simulink model "SimForces2022a"  (R2022a)
settings: Solver=daessc  StartTime=0.0  StopTime=10  FixedStep=0.001  RelTol=1e-4
values from neighbouring files (symbols this model uses):
  Bc1_V = [0;0;0;0;0;0]    [initializeSimulationGP.m]
  D22F = [0;0;0;0;0;0]    [initializeSimulationGP.m]
  filtDV = init2ndOrderLowPassFilter(35*2*pi,1,controller.dT)    [initializeLowPassFilters.m]
  filtEnc = init2ndOrderLowPassFilter(35*2*pi,1,controller.dT)    [initializeLowPassFilters.m]
undefined symbols (not defined in the file or in its folder): aux, B11_r_B11Tc1, B11_V, B11Ftot, B12_r_B12Tc2, B12_Rot_Tc2, B12_U_Tc2, B12_V, B12Ftot, B31_r_B31B41, B31_V, B31FTot, B32_r_B32B42, B32_Rot_B42, B32_U_B42, B32_V, B32FTot, B41_r_B41Tc1, B41_V, B41FTot, B42_r_B42Tc2, B42_Rot_Tc2, B42_U_Tc2, B42_V, B42FTot, B52_r_B52P32, B52_Rot_P32, B52_U_P32, B52_V, B52Ftot, Bc1_r_Bc1B11, Bc1_r_Bc1B31, Bc1FTot, Bc2_r_Bc2B12, Bc2_r_Bc2B32, Bc2_Rot_B12, Bc2_Rot_B32, Bc2_U_B12, Bc2_U_B32, Bc2_V, Bc2Tot, controller, cyl1, cyl2, D22_V, dq1, dq11, dq12, dq2, dq21, dq22, dx1, dx2, dxt2, fc1, fc1r, fc2, fc2r, fct2, fct2r ... (+61)
libraries: sm_lib x32, nesl_utility x20
(part 3 of 7)

== system SimForces2022a/sbVDCController/sbFormAnalyticQuantities/sbRevoluteSegment2 ==
  note: Due to repeatable nature of the calculation process, all the comments in RS1 remain in RS2.
  note: Get inputs...
  note: Process data...
  note: Pass to outputs...
  q2 : Inport
  WRotXRS1 : Inport  Port=2
  velsRS1 : Inport  Port=3
  sbGeomPropRS2 : Subsystem
  sbPosVecsRS2 : Subsystem
  sbRotMatsRS2 : Subsystem
  sbUMatsRS2 : Subsystem
  sbVelsRS2 : Subsystem
  geomPropRS2 : Outport
  WRotXRS2 : Outport  Port=2
  UMatsRS2 : Outport  Port=3
  velsRS2 : Outport  Port=4
  wires:
  [velsRS2] -> velsRS2/1  "velsRS2"
  sbVelsRS2/1(velsRS2) -> [velsRS2]  "velsRS2"
  [WRotXRS1] -> sbRotMatsRS2/2(WRotXRS1)  "WRotXRS1"
  WRotXRS1/1 -> [WRotXRS1]  "WRotXRS1"
  [velsRS1] -> sbVelsRS2/3(velsRS1)  "velsRS1"
  velsRS1/1 -> [velsRS1]  "velsRS1"
  [WRotXRS2] -> WRotXRS2/1  "WRotXRS2"
  sbRotMatsRS2/2(WRotXRS2) -> [WRotXRS2]  "WRotXRS2"
  [UMatsRS2] -> UMatsRS2/1  "UMatsRS2"
  [UMatsRS2] -> sbVelsRS2/2(UMatsRS2)  "UMatsRS2"
  sbUMatsRS2/1(UMatsRS2) -> [UMatsRS2]  "UMatsRS2"
  [rotMatsRS2] -> sbUMatsRS2/2(rotMatsRS2)  "rotMatsRS2"
  [posVecsRS2] -> sbUMatsRS2/1(posVecsRS2)  "posVecsRS2"
  sbPosVecsRS2/1(posVecsRS2) -> [posVecsRS2]  "posVecsRS2"
  q2/1 -> [q2]  "q2"
  sbRotMatsRS2/1(rotMatsRS2) -> [rotMatsRS2]  "rotMatsRS2"
  [geomPropRS2] -> geomPropRS2/1  "geomPropRS2"
  [q2] -> sbGeomPropRS2/1(q2)  "q2"
  sbGeomPropRS2/1(geomPropRS2) -> [geomPropRS2]  "geomPropRS2"
  [geomPropRS2] -> sbPosVecsRS2/1(geomPropRS2)  "geomPropRS2"
  [geomPropRS2] -> sbRotMatsRS2/1(geomPropRS2)  "geomPropRS2"
  [geomPropRS2] -> sbVelsRS2/1(geomPropRS2)  "geomPropRS2"

== system SimForces2022a/sbVDCController/sbFormTotalRequiredForces/sbTotalRequiredForcesPS2 ==
  note: Form new buses...
  note: Pass to outputs...
  note: Process data...
  note: Get inputs...
  note: Select from existing buses...
  note: Calculate total forces in the prismatic segment 2 (PS2).
  velsX : Inport
  WRotX : Inport  Port=2
  Bus Creator1 : BusCreator  Inputs=P22FTot,B52Ftot,P32FTot
  Bus Selector2 : BusSelector  OutputSignals=WRotXRS2.W_Rot_P22,WRotXPS2.W_Rot_B52,WRotXPS2.W_Rot_P32
  Bus Selector3 : BusSelector  OutputSignals=velsRS2.P22_V,velsPS2.B52_V,velsPS2.P32_V
  Constant : Constant  Value=update.thetaB52rNominal
  Constant1 : Constant  Value=update.thetaP22rNominal
  Constant2 : Constant  Value=update.thetaP32rNominal
  Product1 : Product  Multiplication=Matrix(*)
  Product2 : Product  Multiplication=Matrix(*)
  Product3 : Product  Multiplication=Matrix(*)
  Transpose : Math  Operator=transpose
  Transpose1 : Math  Operator=transpose
  Transpose2 : Math  Operator=transpose
  regressorYB52r : MATLAB Function  TreatAsAtomicUnit=on
  regressorYP22r : MATLAB Function  TreatAsAtomicUnit=on
  regressorYP32r : MATLAB Function  TreatAsAtomicUnit=on
  sbFilteredVelocityDerivativeB52 : Subsystem
  sbFilteredVelocityDerivativeP22 : Subsystem
  sbFilteredVelocityDerivativeP32 : Subsystem
  FTotRS2 : Outport
  wires:
  [B52FTot] -> Bus Creator1/2  "B52Ftot"
  Bus Selector3/3 -> [P32V]  "<P32_V>"
  velsX/1 -> [velsX]  "velsX"
  Bus Selector3/2 -> [B52V]  "<B52_V>"
  Bus Selector2/3 -> [WRotP32]  "<W_Rot_P32>"
  WRotX/1 -> [WRotX]  "WRotX"
  [velsX] -> Bus Selector3/1  "velsX"
  Bus Selector2/2 -> [WRotB52]  "<W_Rot_B52>"
  [FTotRS2] -> FTotRS2/1  "FTotRS2"
  [P32FTot] -> Bus Creator1/3  "P32FTot"
  [P22FTot] -> Bus Creator1/1  "P22FTot"
  [WRotX] -> Bus Selector2/1  "WRotX"
  Bus Selector2/1 -> [WRotP22]  "<W_Rot_P22>"
  Bus Selector3/1 -> [P22V]  "<P22_V>"
  Bus Creator1/1 -> [FTotRS2]  "FTotRS2"
  [WRotP32] -> Transpose2/1  "W_Rot_P32"
  [WRotB52] -> Transpose1/1  "W_Rot_B52"
  regressorYP32r/1(YP32r) -> Product3/1  "YP32r"
  regressorYB52r/1(YB52r) -> Product2/1  "YB52r"
  [WRotP22] -> Transpose/1  "W_Rot_P22"
  [P32V] -> sbFilteredVelocityDerivativeP32/1(u)  "P32V"
  Transpose1/1 -> regressorYB52r/3(B52_Rot_W)  "B52_Rot_W"
  Transpose2/1 -> regressorYP32r/3(P32_Rot_W)  "P32_Rot_W"
  sbFilteredVelocityDerivativeP22/1(du) -> regressorYP22r/2(P22dV)  "P22dV"
  Product1/1 -> [P22FTot]  "P22FTot"
  Product3/1 -> [P32FTot]  "P32FTot"
  Product2/1 -> [B52FTot]  "B52FTot"
  sbFilteredVelocityDerivativeB52/1(du) -> regressorYB52r/2(B52dV)  "B52dV"
  [B52V] -> sbFilteredVelocityDerivativeB52/1(u)  "B52V"
  sbFilteredVelocityDerivativeP32/1(du) -> regressorYP32r/2(P32dV)  "P32dV"
  Transpose/1 -> regressorYP22r/3(P22_Rot_W)  "P22_Rot_W"
  [P22V] -> sbFilteredVelocityDerivativeP22/1(u)  "P22V"
  regressorYP22r/1(YP22r) -> Product1/1  "YP22r"
  Constant/1 -> Product2/2  "thetaB52rNominal"
  Constant1/1 -> Product1/2  "thetaP22rNominal"
  Constant2/1 -> Product3/2  "thetaP32rNominal"
  [P32V] -> regressorYP32r/1(P32V)  "P32V"
  [B52V] -> regressorYB52r/1(B52V)  "B52V"
  [P22V] -> regressorYP22r/1(P22V)  "P22V"

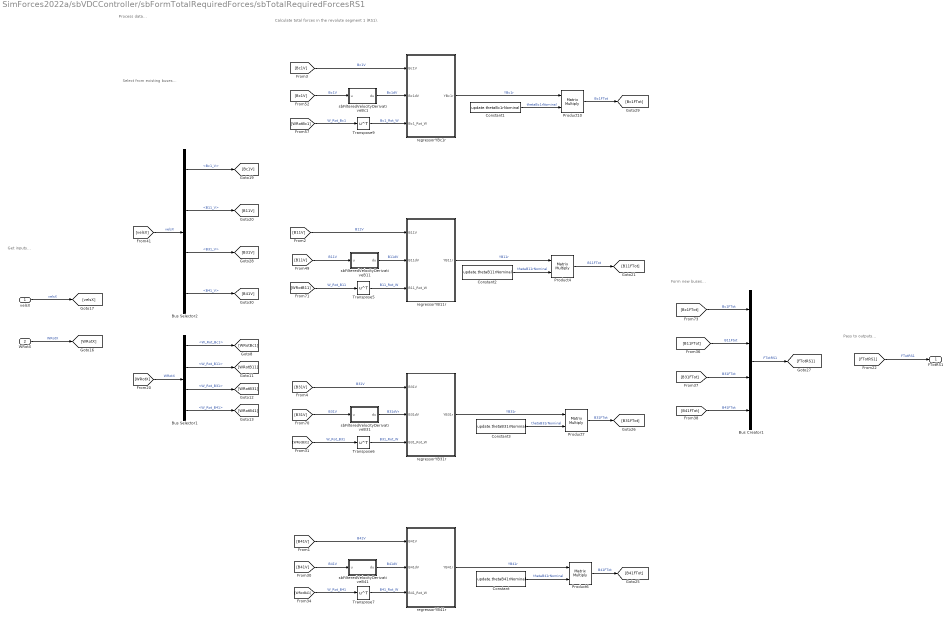
== system SimForces2022a/sbVDCController/sbFormTotalRequiredForces/sbTotalRequiredForcesRS1 ==
  note: Select from existing buses...
  note: Process data...
  note: Get inputs...
  note: Pass to outputs...
  note: Calculate total forces in the revolute segment 1 (RS1).
  note: Form new buses...
  velsX : Inport
  WRotX : Inport  Port=2
  Bus Creator1 : BusCreator  Inputs=Bc1FTot,B11Ftot,B31FTot,B41FTot
  Bus Selector1 : BusSelector  OutputSignals=WRotXRS1.W_Rot_Bc1,WRotXRS1.W_Rot_B11,WRotXRS1.W_Rot_B31,WRotXRS1.W_Rot_B41
  Bus Selector2 : BusSelector  OutputSignals=velsRS1.Bc1_V,velsRS1.B11_V,velsRS1.B31_V,velsRS1.B41_V
  Constant : Constant  Value=update.thetaB41rNominal
  Constant1 : Constant  Value=update.thetaBc1rNominal
  Constant2 : Constant  Value=update.thetaB11rNominal
  Constant3 : Constant  Value=update.thetaB31rNominal
  Product{4,6..7,10} (4 alike) : Product  Multiplication=Matrix(*)
  Transpose{5..7,9} (4 alike) : Math  Operator=transpose
  regressorYB11r : MATLAB Function  TreatAsAtomicUnit=on
  regressorYB31r : MATLAB Function  TreatAsAtomicUnit=on
  regressorYB41r : MATLAB Function  TreatAsAtomicUnit=on
  regressorYBc1r : MATLAB Function  TreatAsAtomicUnit=on
  sbFilteredVelocityDerivativeB11 : Subsystem
  sbFilteredVelocityDerivativeB31 : Subsystem
  sbFilteredVelocityDerivativeB41 : Subsystem
  sbFilteredVelocityDerivativeBc1 : Subsystem
  FTotRS1 : Outport
  wires:
  [FTotRS1] -> FTotRS1/1  "FTotRS1"
  velsX/1 -> [velsX]  "velsX"
  [WRotX] -> Bus Selector1/1  "WRotX"
  WRotX/1 -> [WRotX]  "WRotX"
  Bus Selector1/4 -> [WRotB41]  "<W_Rot_B41>"
  Bus Selector1/2 -> [WRotB11]  "<W_Rot_B11>"
  Bus Selector1/1 -> [WRotBc1]  "<W_Rot_Bc1>"
  Bus Selector1/3 -> [WRotB31]  "<W_Rot_B31>"
  regressorYB31r/1(YB31r) -> Product7/1  "YB31r"
  sbFilteredVelocityDerivativeB31/1(du) -> regressorYB31r/2(B31dV)  "B31dVr"
  [velsX] -> Bus Selector2/1  "velsX"
  sbFilteredVelocityDerivativeB41/1(du) -> regressorYB41r/2(B41dV)  "B41dV"
  Bus Creator1/1 -> [FTotRS1]  "FTotRS1"
  Product10/1 -> [Bc1FTot]  "Bc1FTot"
  [Bc1FTot] -> Bus Creator1/1  "Bc1FTot"
  [WRotB31] -> Transpose6/1  "W_Rot_B31"
  [B41FTot] -> Bus Creator1/4  "B41FTot"
  Bus Selector2/1 -> [Bc1V]  "<Bc1_V>"
  [B31FTot] -> Bus Creator1/3  "B31FTot"
  [WRotBc1] -> Transpose9/1  "W_Rot_Bc1"
  Transpose5/1 -> regressorYB11r/3(B11_Rot_W)  "B11_Rot_W"
  [WRotB11] -> Transpose5/1  "W_Rot_B11"
  Bus Selector2/2 -> [B11V]  "<B11_V>"
  Bus Selector2/4 -> [B41V]  "<B41_V>"
  regressorYBc1r/1(YBc1r) -> Product10/1  "YBc1r"
  regressorYB11r/1(YB11r) -> Product4/1  "YB11r"
  regressorYB41r/1(YB41r) -> Product6/1  "YB41r"
  [WRotB41] -> Transpose7/1  "W_Rot_B41"
  sbFilteredVelocityDerivativeB11/1(du) -> regressorYB11r/2(B11dV)  "B11dV"
  [Bc1V] -> sbFilteredVelocityDerivativeBc1/1(u)  "Bc1V"
  Transpose7/1 -> regressorYB41r/3(B41_Rot_W)  "B41_Rot_W"
  Transpose9/1 -> regressorYBc1r/3(Bc1_Rot_W)  "Bc1_Rot_W"
  [B11FTot] -> Bus Creator1/2  "B11Ftot"
  Product6/1 -> [B41FTot]  "B41FTot"
  Bus Selector2/3 -> [B31V]  "<B31_V>"
  [Bc1V] -> regressorYBc1r/1(Bc1V)  "Bc1V"
  sbFilteredVelocityDerivativeBc1/1(du) -> regressorYBc1r/2(Bc1dV)  "Bc1dV"
  Transpose6/1 -> regressorYB31r/3(B31_Rot_W)  "B31_Rot_W"
  Product4/1 -> [B11FTot]  "B11FTot"
  Product7/1 -> [B31FTot]  "B31FTot"
  Constant/1 -> Product6/2  "thetaB41rNominal"
  Constant3/1 -> Product7/2  "thetaB31rNominal"
  Constant2/1 -> Product4/2  "thetaB11rNominal"
  Constant1/1 -> Product10/2  "thetaBc1rNominal"
  [B41V] -> sbFilteredVelocityDerivativeB41/1(u)  "B41V"
  [B41V] -> regressorYB41r/1(B41V)  "B41V"
  [B11V] -> sbFilteredVelocityDerivativeB11/1(u)  "B11V"
  [B11V] -> regressorYB11r/1(B11V)  "B11V"
  [B31V] -> sbFilteredVelocityDerivativeB31/1(u)  "B31V"
  [B31V] -> regressorYB31r/1(B31V)  "B31V"

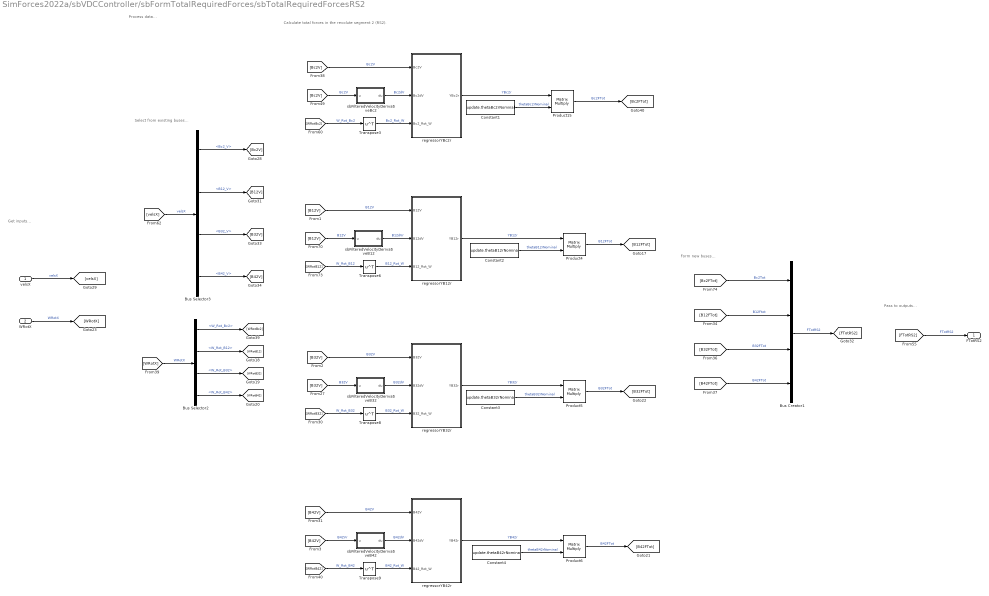
== system SimForces2022a/sbVDCController/sbFormTotalRequiredForces/sbTotalRequiredForcesRS2 ==
  note: Form new buses...
  note: Calculate total forces in the revolute segment 2 (RS2).
  note: Select from existing buses...
  note: Process data...
  note: Pass to outputs...
  note: Get inputs...
  velsX : Inport
  WRotX : Inport  Port=2
  Bus Creator1 : BusCreator  Inputs=Bc2Tot,B12Ftot,B32FTot,B42FTot
  Bus Selector2 : BusSelector  OutputSignals=WRotXRS1.W_Rot_Bc2,WRotXRS2.W_Rot_B12,WRotXRS2.W_Rot_B32,WRotXRS2.W_Rot_B42
  Bus Selector3 : BusSelector  OutputSignals=velsRS2.Bc2_V,velsRS2.B12_V,velsRS2.B32_V,velsRS2.B42_V
  Constant1 : Constant  Value=update.thetaBc2rNominal
  Constant2 : Constant  Value=update.thetaB12rNominal
  Constant3 : Constant  Value=update.thetaB32rNominal
  Constant4 : Constant  Value=update.thetaB42rNominal
  Product{4..6,15} (4 alike) : Product  Multiplication=Matrix(*)
  Transpose{3,6,8..9} (4 alike) : Math  Operator=transpose
  regressorYB12r : MATLAB Function  TreatAsAtomicUnit=on
  regressorYB32r : MATLAB Function  TreatAsAtomicUnit=on
  regressorYB42r : MATLAB Function  TreatAsAtomicUnit=on
  regressorYBc2r : MATLAB Function  TreatAsAtomicUnit=on
  sbFilteredVelocityDerivativeB12 : Subsystem
  sbFilteredVelocityDerivativeB32 : Subsystem
  sbFilteredVelocityDerivativeB42 : Subsystem
  sbFilteredVelocityDerivativeBc2 : Subsystem
  FTotRS2 : Outport
  wires:
  Bus Selector3/1 -> [Bc2V]  "<Bc2_V>"
  Bus Selector2/1 -> [WRotBc2]  "<W_Rot_Bc2>"
  Bus Creator1/1 -> [FTotRS2]  "FTotRS2"
  [B32FTot] -> Bus Creator1/3  "B32FTot"
  [WRotX] -> Bus Selector2/1  "WRotX"
  [FTotRS2] -> FTotRS2/1  "FTotRS2"
  [B42FTot] -> Bus Creator1/4  "B42FTot"
  [Bc2FTot] -> Bus Creator1/1  "Bc2Tot"
  Product5/1 -> [B32FTot]  "B32FTot"
  Bus Selector2/2 -> [WRotB12]  "<W_Rot_B12>"
  Bus Selector2/4 -> [WRotB42]  "<W_Rot_B42>"
  Transpose6/1 -> regressorYB12r/3(B12_Rot_W)  "B12_Rot_W"
  [B32V] -> sbFilteredVelocityDerivativeB32/1(u)  "B32V"
  [WRotB32] -> Transpose8/1  "W_Rot_B32"
  sbFilteredVelocityDerivativeB32/1(du) -> regressorYB32r/2(B32dV)  "B32dV"
  Product15/1 -> [Bc2FTot]  "Bc2FTot"
  [B42V] -> sbFilteredVelocityDerivativeB42/1(u)  "B42Vr"
  Transpose9/1 -> regressorYB42r/3(B42_Rot_W)  "B42_Rot_W"
  Product6/1 -> [B42FTot]  "B42FTot"
  regressorYB32r/1(YB32r) -> Product5/1  "YB32r"
  regressorYBc2r/1(YBc2r) -> Product15/1  "YBc2r"
  regressorYB12r/1(YB12r) -> Product4/1  "YB12r"
  [velsX] -> Bus Selector3/1  "velsX"
  [WRotB42] -> Transpose9/1  "W_Rot_B42"
  regressorYB42r/1(YB42r) -> Product6/1  "YB42r"
  Bus Selector3/4 -> [B42V]  "<B42_V>"
  WRotX/1 -> [WRotX]  "WRotX"
  Transpose8/1 -> regressorYB32r/3(B32_Rot_W)  "B32_Rot_W"
  Bus Selector2/3 -> [WRotB32]  "<W_Rot_B32>"
  [WRotBc2] -> Transpose3/1  "W_Rot_Bc2"
  sbFilteredVelocityDerivativeBc2/1(du) -> regressorYBc2r/2(Bc2dV)  "Bc2dV"
  Product4/1 -> [B12FTot]  "B12FTot"
  [B32V] -> regressorYB32r/1(B32V)  "B32V"
  [WRotB12] -> Transpose6/1  "W_Rot_B12"
  sbFilteredVelocityDerivativeB42/1(du) -> regressorYB42r/2(B42dV)  "B42dV"
  sbFilteredVelocityDerivativeB12/1(du) -> regressorYB12r/2(B12dV)  "B12dVr"
  Bus Selector3/2 -> [B12V]  "<B12_V>"
  Bus Selector3/3 -> [B32V]  "<B32_V>"
  [Bc2V] -> sbFilteredVelocityDerivativeBc2/1(u)  "Bc2V"
  velsX/1 -> [velsX]  "velsX"
  Transpose3/1 -> regressorYBc2r/3(Bc2_Rot_W)  "Bc2_Rot_W"
  [B12FTot] -> Bus Creator1/2  "B12Ftot"
  Constant4/1 -> Product6/2  "thetaB42rNominal"
  Constant3/1 -> Product5/2  "thetaB32rNominal"
  Constant2/1 -> Product4/2  "thetaB12rNominal"
  [Bc2V] -> regressorYBc2r/1(Bc2V)  "Bc2V"
  Constant1/1 -> Product15/2  "thetaBc2rNominal"
  [B12V] -> sbFilteredVelocityDerivativeB12/1(u)  "B12V"
  [B12V] -> regressorYB12r/1(B12V)  "B12V"
  [B42V] -> regressorYB42r/1(B42V)  "B42V"

== system SimForces2022a/sbVDCController/sbFormAnalyticQuantities/sbPrismaticSegment2/sbGeomPropPS2 ==
  note: Get inputs...
  note: Process data...
  note: Pass to outputs...
  xt2 : Inport
  Bus Creator : BusCreator  Inputs=xt2,dxt2
  sbDiscreteDerivative : Subsystem
  geomPropPS2 : Outport
  wires:
  xt2/1 -> [xt2]
  [xt2] -> sbDiscreteDerivative/1(u)  "xt2"
  sbDiscreteDerivative/1(du/dt) -> [dxt2]  "dxt2"
  [xt2] -> Bus Creator/1  "xt2"
  [dxt2] -> Bus Creator/2  "dxt2"
  Bus Creator/1 -> [geomPropPS2]  "geomPropPS2"
  [geomPropPS2] -> geomPropPS2/1  "geomPropPS2"

== system SimForces2022a/sbVDCController/sbFormAnalyticQuantities/sbPrismaticSegment2/sbPosVecsPS2 ==
  note: Get inputs...
  note: Process data...
  note: Pass to outputs...
  xt2 : Inport
  Bus Creator : BusCreator  Inputs=P22_r_P22B52,B52_r_B52P32,P32_r_P32D22
  Constant : Constant  Value=posVec.B52_r_B52P32
  Constant1 : Constant  Value=posVec.P32_r_P32D22
  P22_r_P22B52 : MATLAB Function  TreatAsAtomicUnit=on
  posVecsPS2 : Outport
  wires:
  [rP32D22] -> Bus Creator/3  "P32_r_P32D22"
  Constant1/1 -> [rP32D22]  "P32_r_P32D22"
  [PosVecsS2P] -> posVecsPS2/1
  Bus Creator/1 -> [PosVecsS2P]
  [rB52P32] -> Bus Creator/2  "B52_r_B52P32"
  [rP22B52] -> Bus Creator/1  "P22_r_P22B52"
  Constant/1 -> [rB52P32]  "B52_r_B52P32"
  P22_r_P22B52/1(P22_r_P22B52) -> [rP22B52]  "P22_r_P22B52"
  [xt2] -> P22_r_P22B52/1(xt2)
  xt2/1 -> [xt2]

== system SimForces2022a/sbVDCController/sbFormAnalyticQuantities/sbPrismaticSegment2/sbRotMatsPS2 ==
  note: Process data...
  note: Get inputs...
  note: Pass to outputs...
  WRotXRS2 : Inport
  Bus Creator1 : BusCreator  Inputs=W_Rot_B52,W_Rot_P32,W_Rot_D22
  Bus Creator2 : BusCreator  Inputs=P22_Rot_B52,B52_Rot_P32,P32_Rot_D22
  Bus Selector : BusSelector  OutputSignals=W_Rot_P22
  Constant : Constant  Value=rotMat.P22_Rot_B52
  Constant1 : Constant  Value=rotMat.B52_Rot_P32
  Constant2 : Constant  Value=rotMat.P32_Rot_D22
  Product : Product  Multiplication=Matrix(*)
  Product1 : Product  Multiplication=Matrix(*)
  Product2 : Product  Multiplication=Matrix(*)
  rotMatsPS2 : Outport
  WRotXPS2 : Outport  Port=2
  wires:
  Product2/1 -> [WRotD22]
  [WRotD22] -> Bus Creator1/3  "W_Rot_D22"
  [P32RotD22] -> Bus Creator2/3  "P32_Rot_D22"
  [P32RotD22] -> Product2/2
  [WRotP32] -> Product2/1
  Constant2/1 -> [P32RotD22]  "P32_Rot_D22"
  [rotMatsPS2] -> rotMatsPS2/1  "rotMatsPS2"
  [WRotXPS2] -> WRotXPS2/1  "WRotXPS2"
  Bus Creator1/1 -> [WRotXPS2]  "WRotXPS2"
  Bus Creator2/1 -> [rotMatsPS2]  "rotMatsPS2"
  [WRotXRS2] -> Bus Selector/1  "WRotXRS2"
  WRotXRS2/1 -> [WRotXRS2]  "WRotXRS2"
  Bus Selector/1 -> [WRotP22]  "<W_Rot_P22>"
  [P22RotB52] -> Bus Creator2/1  "P22_Rot_B52"
  [B52RotP32] -> Bus Creator2/2  "B52_Rot_P32"
  [WRotP32] -> Bus Creator1/2  "W_Rot_P32"
  [WRotB52] -> Bus Creator1/1  "W_Rot_B52"
  Product1/1 -> [WRotP32]
  [WRotB52] -> Product1/1
  [B52RotP32] -> Product1/2
  Product/1 -> [WRotB52]
  [P22RotB52] -> Product/2
  [WRotP22] -> Product/1
  Constant1/1 -> [B52RotP32]  "B52_Rot_P32"
  Constant/1 -> [P22RotB52]  "P22_Rot_B52"

== system SimForces2022a/sbVDCController/sbFormAnalyticQuantities/sbPrismaticSegment2/sbUMatsPS2 ==
  note: Get inputs...
  note: Process data...
  note: Pass to outputs...
  posVecsPS2 : Inport
  rotMatsPS2 : Inport  Port=2
  B52_U_P32 : MATLAB Function  TreatAsAtomicUnit=on
  Bus Creator : BusCreator  Inputs=P22_U_B52,B52_U_P32,P32_U_D22
  Bus Selector : BusSelector  OutputSignals=P22_r_P22B52,B52_r_B52P32,P32_r_P32D22
  Bus Selector1 : BusSelector  OutputSignals=P22_Rot_B52,B52_Rot_P32,P32_Rot_D22
  P22_U_B52 : MATLAB Function  TreatAsAtomicUnit=on
  P32_U_D22 : MATLAB Function  TreatAsAtomicUnit=on
  UMatsPS2 : Outport
  wires:
  [P32UD22] -> Bus Creator/3  "P32_U_D22"
  P32_U_D22/1(P32_U_D22) -> [P32UD22]  "P32_U_D22"
  [P32RotD22] -> P32_U_D22/2(P32_Rot_D22)
  [rP32D22] -> P32_U_D22/1(P32_r_P32D22)
  Bus Selector/3 -> [rP32D22]  "<P32_r_P32D22>"
  Bus Selector1/3 -> [P32RotD22]  "<P32_Rot_D22>"
  Bus Creator/1 -> [UMatsS2P]
  [UMatsS2P] -> UMatsPS2/1
  [B52UP32] -> Bus Creator/2  "B52_U_P32"
  [P22UB52] -> Bus Creator/1  "P22_U_B52"
  B52_U_P32/1(B52_U_P32) -> [B52UP32]  "B52_U_P32"
  [rB52P32] -> B52_U_P32/1(B52_r_B52B32)
  [B52RotP32] -> B52_U_P32/2(B52_Rot_B32)
  P22_U_B52/1(P22_U_B52) -> [P22UB52]  "P22_U_B52"
  [P22RotB52] -> P22_U_B52/2(P22_Rot_B52)
  [rP22B52] -> P22_U_B52/1(P22_r_P22B52)
  Bus Selector/2 -> [rB52P32]  "<B52_r_B52P32>"
  Bus Selector1/2 -> [B52RotP32]  "<B52_Rot_P32>"
  Bus Selector1/1 -> [P22RotB52]  "<P22_Rot_B52>"
  Bus Selector/1 -> [rP22B52]  "<P22_r_P22B52>"
  [RotMatsS2P] -> Bus Selector1/1
  [PosVecsS2P] -> Bus Selector/1
  rotMatsPS2/1 -> [RotMatsS2P]
  posVecsPS2/1 -> [PosVecsS2P]

== system SimForces2022a/sbVDCController/sbFormAnalyticQuantities/sbPrismaticSegment2/sbVelsPS2 ==
  note: Get inputs...
  note: Process data...
  note: Pass to outputs...
  geomPropPS2 : Inport
  UMatsPS2 : Inport  Port=2
  velsRS2 : Inport  Port=3
  Bus Creator : BusCreator  Inputs=B52_V,P32_V,D22_V
  Bus Selector : BusSelector  OutputSignals=dxt2
  Bus Selector1 : BusSelector  OutputSignals=P22_V
  Bus Selector2 : BusSelector  OutputSignals=P22_U_B52,B52_U_P32,P32_U_D22
  Gain : Gain  Gain=aux.xf
  Product : Product  Multiplication=Matrix(*)
  Product1 : Product  Multiplication=Matrix(*)
  Product2 : Product  Multiplication=Matrix(*)
  Sum : Sum  Inputs=|++
  Transpose : Math  Operator=transpose
  Transpose1 : Math  Operator=transpose
  Transpose2 : Math  Operator=transpose
  velsPS2 : Outport
  wires:
  [D22V] -> Bus Creator/3  "D22_V"
  Product2/1 -> [D22V]
  Transpose2/1 -> Product2/1
  [P32UG] -> Transpose2/1
  [P32V] -> Product2/2
  Bus Selector2/3 -> [P32UG]  "<P32_U_D22>"
  [velsPS2] -> velsPS2/1  "velsPS2"
  Bus Creator/1 -> [velsPS2]  "velsPS2"
  [B52V] -> Bus Creator/1  "B52_V"
  [P32V] -> Bus Creator/2  "P32_V"
  Product1/1 -> [P32V]
  [B52UP32] -> Transpose1/1
  Transpose1/1 -> Product1/1
  [B52V] -> Product1/2
  Transpose/1 -> Product/1
  [P22UB52] -> Transpose/1
  [P22V] -> Product/2
  Product/1 -> Sum/2
  Gain/1 -> Sum/1
  Bus Selector2/2 -> [B52UP32]  "<B52_U_P32>"
  Bus Selector2/1 -> [P22UB52]  "<P22_U_B52>"
  [UMatsS2P] -> Bus Selector2/1  "UMatsPS2"
  Sum/1 -> [B52V]
  [dxt2] -> Gain/1
  Bus Selector1/1 -> [P22V]  "<P22_V>"
  UMatsPS2/1 -> [UMatsS2P]  "UMatsPS2"
  [velsRS2] -> Bus Selector1/1  "velsRS2"
  velsRS2/1 -> [velsRS2]  "velsRS2"
  geomPropPS2/1 -> [geomPropPS2]  "geomPropPS2"
  [geomPropPS2] -> Bus Selector/1  "geomPropPS2"
  Bus Selector/1 -> [dxt2]  "<dxt2>"

== system SimForces2022a/sbVDCController/sbFormAnalyticQuantities/sbRevoluteSegment1/sbGeomPropRS1 ==
  note: Calculate lift piston velocity per (21).
  note: Calculate angle q1 derivative numerically.
  note: Calculate q12 angle value per (20).
  note: Calculate q11 angle value per (19).
  note: Calculate lift piston stroke per (18).
  note: Create new buses...
  note: Process data...
  note: Pass to outputs...
  note: Get inputs...
  note: Calculate q11 angle velocity per (22).
  note: Calculate q12 angle velocity per (23).
  q1 : Inport
  Bus Creator : BusCreator  Inputs=q1,x1,q11,q12,dq1,dx1,dq11,dq12
  sbLiftPistonStroke : Subsystem
  sbLiftPistonVelocity : Subsystem
  sbq11AngleValue : Subsystem
  sbq11AngleVelocity : Subsystem
  sbq12AngleRate : Subsystem
  sbq12AngleValue : Subsystem
  sbq1AngleRate : Subsystem
  geomPropRS1 : Outport
  wires:
  [q12] -> sbq12AngleRate/2(q12)  "q12"
  [x1] -> sbq12AngleRate/1(x1)  "x1"
  [dx1] -> sbq12AngleRate/3(dx1)  "dx1"
  sbq12AngleRate/1(dq12) -> [dq12]  "dq12"
  sbq11AngleVelocity/1(dq11) -> [dq11]  "dq11"
  [q11] -> sbq11AngleVelocity/2(q11)  "q11"
  [x1] -> sbq11AngleVelocity/1(x1)  "x1"
  [dx1] -> sbq11AngleVelocity/3(dx1)  "dx1"
  sbLiftPistonVelocity/1(dx1) -> [dx1]  "dx1"
  [q1] -> sbLiftPistonVelocity/3(q1)  "q1"
  [x1] -> sbLiftPistonVelocity/2(x1)  "x1"
  [dq1] -> sbLiftPistonVelocity/1(dq1)  "dq1"
  sbq1AngleRate/1(dq1) -> [dq1]  "dq1"
  [q1] -> sbq1AngleRate/1(q1)  "q1"
  [geomPropRS1] -> geomPropRS1/1  "geomPropRS1"
  Bus Creator/1 -> [geomPropRS1]  "geomPropRS1"
  [dq11] -> Bus Creator/7  "dq11"
  [dq12] -> Bus Creator/8  "dq12"
  [dx1] -> Bus Creator/6  "dx1"
  [q11] -> Bus Creator/3  "q11"
  sbq11AngleValue/1(q11) -> [q11]  "q11"
  [x1] -> Bus Creator/2  "x1"
  [q1] -> Bus Creator/1  "q1"
  [q12] -> Bus Creator/4  "q12"
  sbq12AngleValue/1(q12) -> [q12]  "q12"
  [dq1] -> Bus Creator/5  "dq1"
  [x1] -> sbq12AngleValue/1(x1)  "x1"
  [x1] -> sbq11AngleValue/1(x1)  "x1"
  sbLiftPistonStroke/1(x1) -> [x1]  "x1"
  [q1] -> sbLiftPistonStroke/1(q1)  "q1"
  q1/1 -> [q1]  "q1"

== system SimForces2022a/sbVDCController/sbFormAnalyticQuantities/sbRevoluteSegment1/sbPosVecsRS1 ==
  note: Get inputs...
  note: Form time-varying position vectors...
  note: Process data...
  note: Create new buses...
  note: Pass to outputs...
  note: Select from existing buses...
  geomPropRS1 : Inport
  B11_r_B11Tc1 : Constant  Value=posVec.B11_r_B11Tc1
  B31_r_B31B41 : MATLAB Function  TreatAsAtomicUnit=on
  B41_r_B41Tc1 : Constant  Value=posVec.B41_r_B41Tc1
  Bc1_r_Bc1B11 : Constant  Value=posVec.Bc1_r_Bc1B11
  Bc1_r_Bc1B31 : Constant  Value=posVec.Bc1_r_Bc1B31
  Bus Creator : BusCreator  Inputs=Tc1_r_Tc1Bc2,B41_r_B41Tc1,B31_r_B31B41,Bc1_r_Bc1B31,B11_r_B11Tc1,Bc1_r_Bc1B11,W_r_WBc1
  Bus Selector : BusSelector  OutputSignals=x1
  Tc1_r_Tc1Bc2 : Constant  Value=posVec.Tc1_r_Tc1Bc2
  W_r_WBc1 : Constant  Value=posVec.W_r_WBc1
  posVecsRS1 : Outport
  wires:
  W_r_WBc1/1 -> [rWBc1]  "W_r_WBc1"
  [rWBc1] -> Bus Creator/7  "W_r_WBc1"
  [posVecsRS1] -> posVecsRS1/1  "posVecsRS1"
  [x1] -> B31_r_B31B41/1(x1)  "x1"
  Bus Selector/1 -> [x1]  "<x1>"
  [rBc1B11] -> Bus Creator/6  "Bc1_r_Bc1B11"
  [rB11Tc1] -> Bus Creator/5  "B11_r_B11Tc1"
  [rBc1B31] -> Bus Creator/4  "Bc1_r_Bc1B31"
  Bc1_r_Bc1B11/1 -> [rBc1B11]  "Bc1_r_Bc1B11"
  B11_r_B11Tc1/1 -> [rB11Tc1]  "B11_r_B11Tc1"
  Bc1_r_Bc1B31/1 -> [rBc1B31]  "Bc1_r_Bc1B31"
  [rB31B41] -> Bus Creator/3  "B31_r_B31B41"
  B31_r_B31B41/1(B31_r_B31B41) -> [rB31B41]  "B31_r_B31B41"
  [rB41Tc1] -> Bus Creator/2  "B41_r_B41Tc1"
  B41_r_B41Tc1/1 -> [rB41Tc1]  "B41_r_B41Tc1"
  [rTc1Bc2] -> Bus Creator/1  "Tc1_r_Tc1Bc2"
  Tc1_r_Tc1Bc2/1 -> [rTc1Bc2]  "Tc1_r_Tc1Bc2"
  [geomPropRS1] -> Bus Selector/1  "geomPropRS1"
  geomPropRS1/1 -> [geomPropRS1]  "geomPropRS1"
  Bus Creator/1 -> [posVecsRS1]  "posVecsRS1"

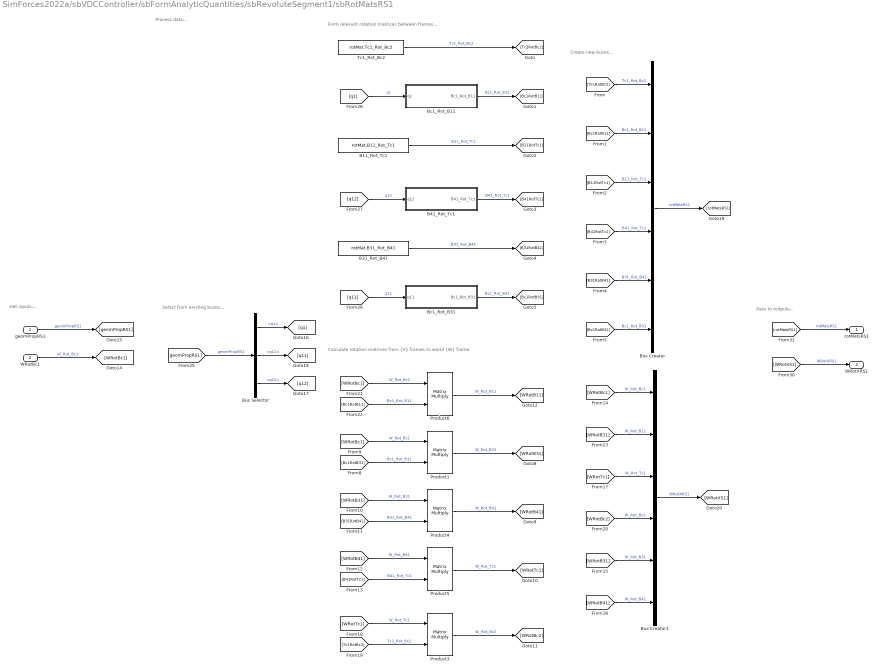
== system SimForces2022a/sbVDCController/sbFormAnalyticQuantities/sbRevoluteSegment1/sbRotMatsRS1 ==
  note: Calculate rotation matrices from {X} frames to world {W} frame
  note: Form relevant rotation matrices between frames...
  note: Select from existing buses...
  note: Process data...
  note: Get inputs...
  note: Pass to outputs...
  note: Create new buses...
  geomPropRS1 : Inport
  WRotBc1 : Inport  Port=2
  B11_Rot_Tc1 : Constant  Value=rotMat.B11_Rot_Tc1
  B31_Rot_B41 : Constant  Value=rotMat.B31_Rot_B41
  B41_Rot_Tc1 : MATLAB Function  TreatAsAtomicUnit=on
  Bc1_Rot_B11 : MATLAB Function  TreatAsAtomicUnit=on
  Bc1_Rot_B31 : MATLAB Function  TreatAsAtomicUnit=on
  Bus Creator : BusCreator  Inputs=6
  Bus Creator1 : BusCreator  Inputs=W_Rot_Bc1,W_Rot_B11,W_Rot_Tc1,W_Rot_Bc2,W_Rot_B31,W_Rot_B41
  Bus Selector : BusSelector  OutputSignals=q1,q11,q12
  Product{1,3..6} (5 alike) : Product  Multiplication=Matrix(*)
  Tc1_Rot_Bc2 : Constant  Value=rotMat.Tc1_Rot_Bc2
  rotMatsRS1 : Outport
  WRotXRS1 : Outport  Port=2
  wires:
  [rotMatsRS1] -> rotMatsRS1/1  "rotMatsRS1"
  [WRotXS1] -> WRotXRS1/1  "WRotXRS1"
  Bus Creator1/1 -> [WRotXS1]  "WRotXRS1"
  Bus Creator/1 -> [rotMatsRS1]  "rotMatsRS1"
  [q11] -> Bc1_Rot_B31/1(q11)  "q11"
  [q12] -> B41_Rot_Tc1/1(q12)  "q12"
  [q1] -> Bc1_Rot_B11/1(q1)  "q1"
  Bus Selector/2 -> [q11]  "<q11>"
  Bus Selector/3 -> [q12]  "<q12>"
  Bus Selector/1 -> [q1]  "<q1>"
  [geomPropRS1] -> Bus Selector/1  "geomPropRS1"
  geomPropRS1/1 -> [geomPropRS1]  "geomPropRS1"
  WRotBc1/1 -> [WRotBc1]  "W_Rot_Bc1"
  [WRotTc1] -> Bus Creator1/3  "W_Rot_Tc1"
  [WRotBc2] -> Bus Creator1/4  "W_Rot_Bc2"
  [WRotB31] -> Bus Creator1/5  "W_Rot_B31"
  [WRotB41] -> Bus Creator1/6  "W_Rot_B41"
  [WRotBc1] -> Bus Creator1/1  "W_Rot_Bc1"
  [WRotB11] -> Bus Creator1/2  "W_Rot_B11"
  Product6/1 -> [WRotB11]  "W_Rot_B11"
  [Bc1RotB11] -> Product6/2  "Bc1_Rot_B11"
  [WRotBc1] -> Product6/1  "W_Rot_Bc1"
  Product3/1 -> [WRotBc2]  "W_Rot_Bc2"
  [Tc1RotBc2] -> Product3/2  "Tc1_Rot_Bc2"
  [WRotTc1] -> Product3/1  "W_Rot_Tc1"
  [WRotB41] -> Product5/1  "W_Rot_B41"
  [B41RotTc1] -> Product5/2  "B41_Rot_Tc1"
  Product5/1 -> [WRotTc1]  "W_Rot_Tc1"
  Product4/1 -> [WRotB41]  "W_Rot_B41"
  [B31RotB41] -> Product4/2  "B31_Rot_B41"
  [WRotB31] -> Product4/1  "W_Rot_B31"
  Product1/1 -> [WRotB31]  "W_Rot_B31"
  [Bc1RotB31] -> Product1/2  "Bc1_Rot_B31"
  [WRotBc1] -> Product1/1  "W_Rot_Bc1"
  [Bc1RotB31] -> Bus Creator/6  "Bc1_Rot_B31"
  Bc1_Rot_B31/1(Bc1_Rot_B31) -> [Bc1RotB31]  "Bc1_Rot_B31"
  [B31RotB41] -> Bus Creator/5  "B31_Rot_B41"
  B31_Rot_B41/1 -> [B31RotB41]  "B31_Rot_B41"
  [B41RotTc1] -> Bus Creator/4  "B41_Rot_Tc1"
  B41_Rot_Tc1/1(B41_Rot_Tc1) -> [B41RotTc1]  "B41_Rot_Tc1"
  B11_Rot_Tc1/1 -> [B11RotTc1]  "B11_Rot_Tc1"
  [B11RotTc1] -> Bus Creator/3  "B11_Rot_Tc1"
  Bc1_Rot_B11/1(Bc1_Rot_B11) -> [Bc1RotB11]  "Bc1_Rot_B11"
  [Bc1RotB11] -> Bus Creator/2  "Bc1_Rot_B11"
  Tc1_Rot_Bc2/1 -> [Tc1RotBc2]  "Tc1_Rot_Bc2"
  [Tc1RotBc2] -> Bus Creator/1  "Tc1_Rot_Bc2"

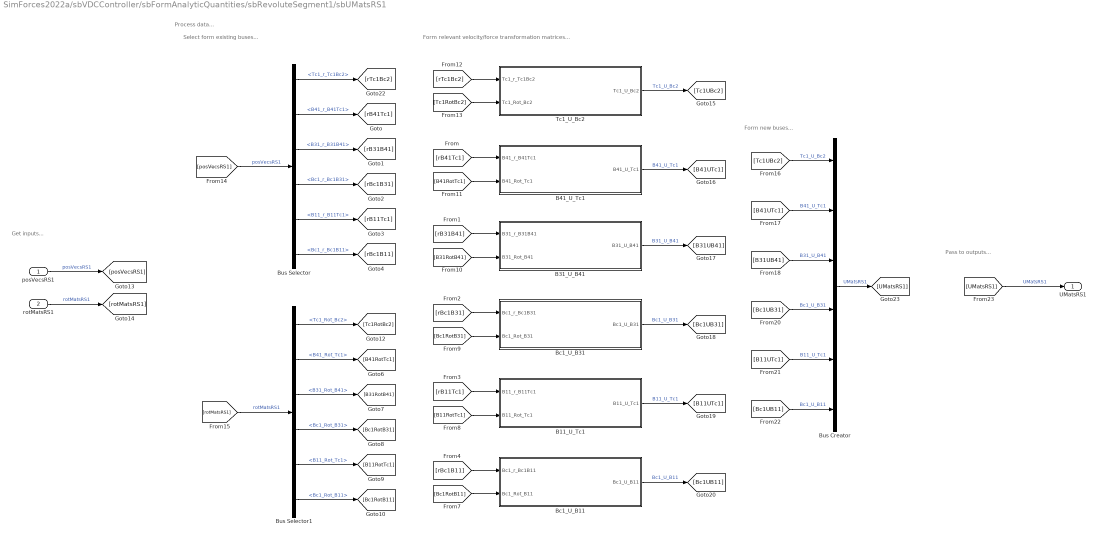
== system SimForces2022a/sbVDCController/sbFormAnalyticQuantities/sbRevoluteSegment1/sbUMatsRS1 ==
  note: Select form existing buses...
  note: Form relevant velocity/force transformation matrices...
  note: Process data...
  note: Form new buses...
  note: Pass to outputs...
  note: Get inputs...
  posVecsRS1 : Inport
  rotMatsRS1 : Inport  Port=2
  B11_U_Tc1 : MATLAB Function  TreatAsAtomicUnit=on
  B31_U_B41 : MATLAB Function  TreatAsAtomicUnit=on
  B41_U_Tc1 : MATLAB Function  TreatAsAtomicUnit=on
  Bc1_U_B11 : MATLAB Function  TreatAsAtomicUnit=on
  Bc1_U_B31 : MATLAB Function  TreatAsAtomicUnit=on
  Bus Creator : BusCreator  Inputs=6
  Bus Selector : BusSelector  OutputSignals=Tc1_r_Tc1Bc2,B41_r_B41Tc1,B31_r_B31B41,Bc1_r_Bc1B31,B11_r_B11Tc1,Bc1_r_Bc1B11
  Bus Selector1 : BusSelector  OutputSignals=Tc1_Rot_Bc2,B41_Rot_Tc1,B31_Rot_B41,Bc1_Rot_B31,B11_Rot_Tc1,Bc1_Rot_B11
  Tc1_U_Bc2 : MATLAB Function  TreatAsAtomicUnit=on
  UMatsRS1 : Outport
  wires:
  [UMatsRS1] -> UMatsRS1/1  "UMatsRS1"
  [Bc1UB11] -> Bus Creator/6  "Bc1_U_B11"
  [B11UTc1] -> Bus Creator/5  "B11_U_Tc1"
  [Bc1UB31] -> Bus Creator/4  "Bc1_U_B31"
  Bc1_U_B11/1(Bc1_U_B11) -> [Bc1UB11]  "Bc1_U_B11"
  B11_U_Tc1/1(B11_U_Tc1) -> [B11UTc1]  "B11_U_Tc1"
  Bc1_U_B31/1(Bc1_U_B31) -> [Bc1UB31]  "Bc1_U_B31"
  [B31UB41] -> Bus Creator/3  "B31_U_B41"
  B31_U_B41/1(B31_U_B41) -> [B31UB41]  "B31_U_B41"
  [B41UTc1] -> Bus Creator/2  "B41_U_Tc1"
  B41_U_Tc1/1(B41_U_Tc1) -> [B41UTc1]  "B41_U_Tc1"
  [Tc1UBc2] -> Bus Creator/1  "Tc1_U_Bc2"
  Tc1_U_Bc2/1(Tc1_U_Bc2) -> [Tc1UBc2]  "Tc1_U_Bc2"
  [rotMatsRS1] -> Bus Selector1/1  "rotMatsRS1"
  rotMatsRS1/1 -> [rotMatsRS1]  "rotMatsRS1"
  [posVecsRS1] -> Bus Selector/1  "posVecsRS1"
  posVecsRS1/1 -> [posVecsRS1]  "posVecsRS1"
  Bus Creator/1 -> [UMatsRS1]  "UMatsRS1"
  [rTc1Bc2] -> Tc1_U_Bc2/1(Tc1_r_Tc1Bc2)
  [Tc1RotBc2] -> Tc1_U_Bc2/2(Tc1_Rot_Bc2)
  Bus Selector/1 -> [rTc1Bc2]  "<Tc1_r_Tc1Bc2>"
  Bus Selector1/1 -> [Tc1RotBc2]  "<Tc1_Rot_Bc2>"
  [B41RotTc1] -> B41_U_Tc1/2(B41_Rot_Tc1)
  [B31RotB41] -> B31_U_B41/2(B31_Rot_B41)
  [Bc1RotB31] -> Bc1_U_B31/2(Bc1_Rot_B31)
  [B11RotTc1] -> B11_U_Tc1/2(B11_Rot_Tc1)
  [Bc1RotB11] -> Bc1_U_B11/2(Bc1_Rot_B11)
  Bus Selector1/6 -> [Bc1RotB11]  "<Bc1_Rot_B11>"
  Bus Selector1/5 -> [B11RotTc1]  "<B11_Rot_Tc1>"
  Bus Selector1/4 -> [Bc1RotB31]  "<Bc1_Rot_B31>"
  Bus Selector1/3 -> [B31RotB41]  "<B31_Rot_B41>"
  Bus Selector1/2 -> [B41RotTc1]  "<B41_Rot_Tc1>"
  [rB31B41] -> B31_U_B41/1(B31_r_B31B41)
  [rBc1B31] -> Bc1_U_B31/1(Bc1_r_Bc1B31)
  [rB11Tc1] -> B11_U_Tc1/1(B11_r_B11Tc1)
  [rBc1B11] -> Bc1_U_B11/1(Bc1_r_Bc1B11)
  Bus Selector/6 -> [rBc1B11]  "<Bc1_r_Bc1B11>"
  Bus Selector/4 -> [rBc1B31]  "<Bc1_r_Bc1B31>"
  Bus Selector/5 -> [rB11Tc1]  "<B11_r_B11Tc1>"
  Bus Selector/3 -> [rB31B41]  "<B31_r_B31B41>"
  [rB41Tc1] -> B41_U_Tc1/1(B41_r_B41Tc1)
  Bus Selector/2 -> [rB41Tc1]  "<B41_r_B41Tc1>"

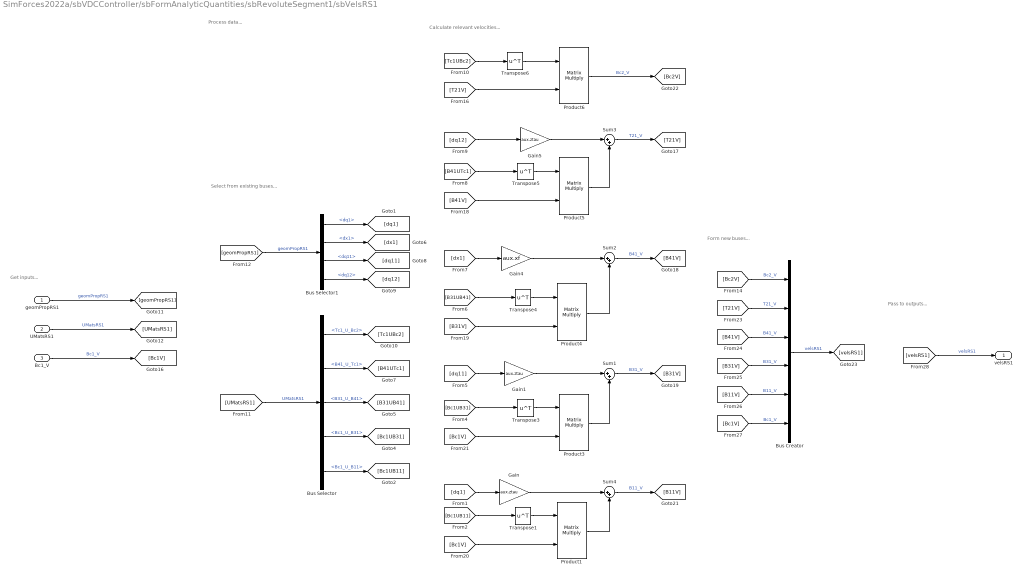
== system SimForces2022a/sbVDCController/sbFormAnalyticQuantities/sbRevoluteSegment1/sbVelsRS1 ==
  note: Get inputs...
  note: Select from existing buses...
  note: Calculate relevant velocities...
  note: Form new buses...
  note: Pass to outputs...
  note: Process data...
  geomPropRS1 : Inport
  UMatsRS1 : Inport  Port=2
  Bc1_V : Inport  Port=3
  Bus Creator : BusCreator  Inputs=Bc2_V,T21_V,B41_V,B31_V,B11_V,Bc1_V
  Bus Selector : BusSelector  OutputSignals=Tc1_U_Bc2,B41_U_Tc1,B31_U_B41,Bc1_U_B31,Bc1_U_B11
  Bus Selector1 : BusSelector  OutputSignals=dq1,dx1,dq11,dq12
  Gain : Gain  Gain=aux.ztau
  Gain1 : Gain  Gain=aux.ztau
  Gain4 : Gain  Gain=aux.xf
  Gain5 : Gain  Gain=aux.ztau
  Product{1,3..6} (5 alike) : Product  Multiplication=Matrix(*)
  Sum{1..4} (4 alike) : Sum  Inputs=|++
  Transpose{1,3..6} (5 alike) : Math  Operator=transpose
  velsRS1 : Outport
  wires:
  [velsRS1] -> velsRS1/1  "velsRS1"
  Bus Creator/1 -> [velsRS1]  "velsRS1"
  [Bc1V] -> Bus Creator/6  "Bc1_V"
  [B11V] -> Bus Creator/5  "B11_V"
  [B31V] -> Bus Creator/4  "B31_V"
  [B41V] -> Bus Creator/3  "B41_V"
  [T21V] -> Bus Creator/2  "T21_V"
  [Bc2V] -> Bus Creator/1  "Bc2_V"
  Product6/1 -> [Bc2V]  "Bc2_V"
  Sum4/1 -> [B11V]  "B11_V"
  [Bc1V] -> Product3/2
  [Bc1V] -> Product1/2
  [B31V] -> Product4/2
  Sum1/1 -> [B31V]  "B31_V"
  [B41V] -> Product5/2
  Sum2/1 -> [B41V]  "B41_V"
  Sum3/1 -> [T21V]  "T21_V"
  [T21V] -> Product6/2
  Bc1_V/1 -> [Bc1V]  "Bc1_V"
  [geomPropRS1] -> Bus Selector1/1  "geomPropRS1"
  [UMatsRS1] -> Bus Selector/1  "UMatsRS1"
  UMatsRS1/1 -> [UMatsRS1]  "UMatsRS1"
  geomPropRS1/1 -> [geomPropRS1]  "geomPropRS1"
  Transpose6/1 -> Product6/1
  [Tc1UBc2] -> Transpose6/1
  Bus Selector/1 -> [Tc1UBc2]  "<Tc1_U_Bc2>"
  [dq12] -> Gain5/1
  Bus Selector1/3 -> [dq11]  "<dq11>"
  Bus Selector1/4 -> [dq12]  "<dq12>"
  Transpose5/1 -> Product5/1
  [B41UTc1] -> Transpose5/1
  Bus Selector/2 -> [B41UTc1]  "<B41_U_Tc1>"
  [dx1] -> Gain4/1
  Bus Selector1/2 -> [dx1]  "<dx1>"
  [B31UB41] -> Transpose4/1
  Transpose4/1 -> Product4/1
  Bus Selector/3 -> [B31UB41]  "<B31_U_B41>"
  [dq11] -> Gain1/1
  Product3/1 -> Sum1/2
  [Bc1UB31] -> Transpose3/1
  Transpose3/1 -> Product3/1
  Bus Selector/4 -> [Bc1UB31]  "<Bc1_U_B31>"
  [Bc1UB11] -> Transpose1/1
  Bus Selector/5 -> [Bc1UB11]  "<Bc1_U_B11>"
  [dq1] -> Gain/1
  Bus Selector1/1 -> [dq1]  "<dq1>"
  Transpose1/1 -> Product1/1
  Product5/1 -> Sum3/2
  Gain4/1 -> Sum2/1
  Product4/1 -> Sum2/2
  Gain/1 -> Sum4/1
  Gain5/1 -> Sum3/1
  Gain1/1 -> Sum1/1
  Product1/1 -> Sum4/2

== system SimForces2022a/sbVDCController/sbFormAnalyticQuantities/sbRevoluteSegment2/sbGeomPropRS2 ==
  note: Get inputs...
  note: Process data...
  note: Pass to outputs...
  q2 : Inport
  Bus Creator : BusCreator  Inputs=q2,x2,q21,q22,dq2,dx2,dq21,dq22
  sbTiltPistonStroke : Subsystem
  sbTiltPistonVelocity : Subsystem
  sbq21AngleRate : Subsystem
  sbq21AngleValue : Subsystem
  sbq22AngleRate : Subsystem
  sbq22AngleValue : Subsystem
  sbq2AngleRate : Subsystem
  geomPropRS2 : Outport
  wires:
  [dx2] -> sbq22AngleRate/3(dx2)  "dx2"
  [q22] -> sbq22AngleRate/2(q22)  "q22"
  [x2] -> sbq22AngleRate/1(x2)  "x2"
  sbq22AngleRate/1(dq22) -> [dq22]  "dq22"
  [dx2] -> sbq21AngleRate/3(dx2)  "dx2"
  [q21] -> sbq21AngleRate/2(q21)  "q21"
  [x2] -> sbq21AngleRate/1(x2)  "x2"
  [geomPropRS2] -> geomPropRS2/1  "geomPropRS2"
  Bus Creator/1 -> [geomPropRS2]  "geomPropRS2"
  [q2] -> sbTiltPistonVelocity/3(q2)  "q2"
  [x2] -> sbTiltPistonVelocity/2(x2)  "x2"
  [dq2] -> sbTiltPistonVelocity/1(dq2)  "dq2"
  sbTiltPistonVelocity/1(dx2) -> [dx2]  "dx2"
  [q2] -> sbq2AngleRate/1(q2)  "q2"
  sbq2AngleRate/1(dq2) -> [dq2]  "dq2"
  [dq22] -> Bus Creator/8  "dq22"
  [dq21] -> Bus Creator/7  "dq21"
  sbq21AngleRate/1(dq21) -> [dq21]  "dq21"
  [q22] -> Bus Creator/4  "q22"
  sbq22AngleValue/1(q22) -> [q22]  "q22"
  [dx2] -> Bus Creator/6  "dx2"
  [x2] -> Bus Creator/2  "x2"
  [q2] -> Bus Creator/1  "q2"
  [q21] -> Bus Creator/3  "q21"
  sbq21AngleValue/1(q21) -> [q21]  "q21"
  [dq2] -> Bus Creator/5  "dq2"
  [x2] -> sbq22AngleValue/1(x2)  "x2"
  [x2] -> sbq21AngleValue/1(x2)  "x2"
  sbTiltPistonStroke/1(x2) -> [x2]  "x2"
  [q2] -> sbTiltPistonStroke/1(q2)  "q2"
  q2/1 -> [q2]  "q2"

== system SimForces2022a/sbVDCController/sbFormAnalyticQuantities/sbRevoluteSegment2/sbPosVecsRS2 ==
  note: Get inputs...
  note: Process data...
  note: Pass to outputs...
  geomPropRS2 : Inport
  B12_r_B12Tc2 : Constant  Value=posVec.B12_r_B12Tc2
  B32_r_B32B42 : MATLAB Function  TreatAsAtomicUnit=on
  B42_r_B42Tc2 : Constant  Value=posVec.B42_r_B42Tc2
  Bc2_r_Bc2B12 : Constant  Value=posVec.Bc2_r_Bc2B12
  Bc2_r_Bc2B32 : Constant  Value=posVec.Bc2_r_Bc2B32
  Bus Creator : BusCreator  Inputs=Tc2_r_Tc2P22,B42_r_B42Tc2,B32_r_B32B42,Bc2_r_Bc2B32,B12_r_B12Tc2,Bc2_r_Bc2B12
  Bus Selector : BusSelector  OutputSignals=x2
  Tc2_r_Tc2P22 : Constant  Value=posVec.Tc2_r_Tc2P22
  posVecsRS2 : Outport
  wires:
  [posVecsRS2] -> posVecsRS2/1  "posVecsRS2"
  Bus Creator/1 -> [posVecsRS2]  "posVecsRS2"
  [rB42Tc2] -> Bus Creator/2  "B42_r_B42Tc2"
  [rB32B42] -> Bus Creator/3  "B32_r_B32B42"
  [rBc2B32] -> Bus Creator/4  "Bc2_r_Bc2B32"
  [rB12Tc2] -> Bus Creator/5  "B12_r_B12Tc2"
  [rBc2B12] -> Bus Creator/6  "Bc2_r_Bc2B12"
  [rTc2P22] -> Bus Creator/1  "Tc2_r_Tc2P22"
  Bc2_r_Bc2B12/1 -> [rBc2B12]  "Bc2_r_Bc2B12"
  B12_r_B12Tc2/1 -> [rB12Tc2]  "B12_r_B12Tc2"
  Bc2_r_Bc2B32/1 -> [rBc2B32]  "Bc2_r_Bc2B32"
  B32_r_B32B42/1(B32_r_B32B42) -> [rB32B42]  "B32_r_B32B42"
  B42_r_B42Tc2/1 -> [rB42Tc2]  "B42_r_B42Tc2"
  Tc2_r_Tc2P22/1 -> [rTc2P22]  "Tc2_r_Tc2P22"
  [geomPropRS2] -> Bus Selector/1  "geomPropRS2"
  geomPropRS2/1 -> [geomPropRS2]  "geomPropRS2"
  Bus Selector/1 -> B32_r_B32B42/1(x2)  "<x2>"

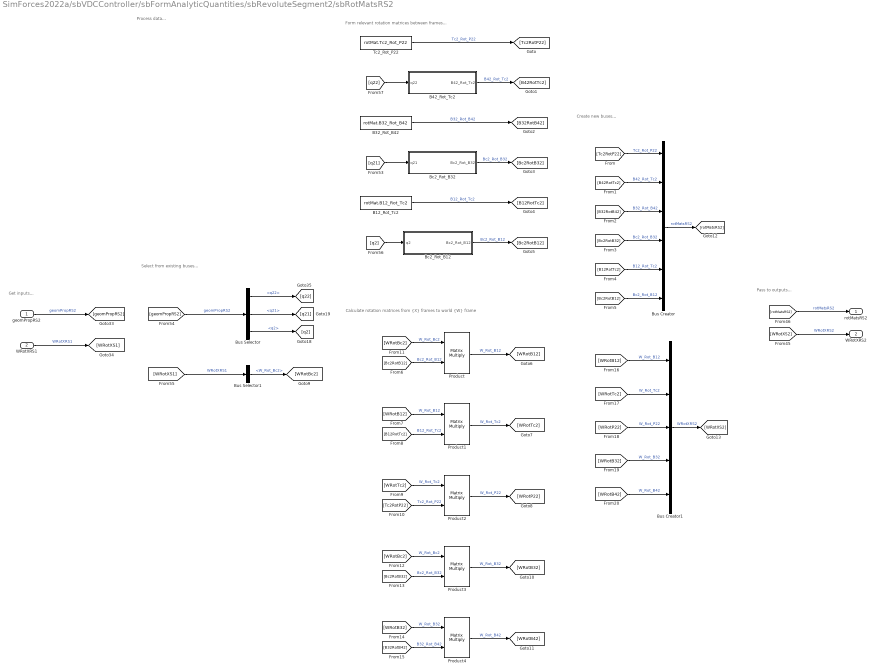
== system SimForces2022a/sbVDCController/sbFormAnalyticQuantities/sbRevoluteSegment2/sbRotMatsRS2 ==
  note: Calculate rotation matrices from {X} frames to world {W} frame
  note: Select from existing buses...
  note: Create new buses...
  note: Form relevant rotation matrices between frames...
  note: Process data...
  note: Get inputs...
  note: Pass to outputs...
  geomPropRS2 : Inport
  WRotXRS1 : Inport  Port=2
  B12_Rot_Tc2 : Constant  Value=rotMat.B12_Rot_Tc2
  B32_Rot_B42 : Constant  Value=rotMat.B32_Rot_B42
  B42_Rot_Tc2 : MATLAB Function  TreatAsAtomicUnit=on
  Bc2_Rot_B12 : MATLAB Function  TreatAsAtomicUnit=on
  Bc2_Rot_B32 : MATLAB Function  TreatAsAtomicUnit=on
  Bus Creator : BusCreator  Inputs=Tc2_Rot_P22,B42_Rot_Tc2,B32_Rot_B42,Bc2_Rot_B32,B12_Rot_Tc2,Bc2_Rot_B12
  Bus Creator1 : BusCreator  Inputs=W_Rot_B12,W_Rot_Tc2,W_Rot_P22,W_Rot_B32,W_Rot_B42
  Bus Selector : BusSelector  OutputSignals=q22,q21,q2
  Bus Selector1 : BusSelector  OutputSignals=W_Rot_Bc2
  Product{,1..4} (5 alike) : Product  Multiplication=Matrix(*)
  Tc2_Rot_P22 : Constant  Value=rotMat.Tc2_Rot_P22
  rotMatsRS2 : Outport
  WRotXRS2 : Outport  Port=2
  wires:
  [q22] -> B42_Rot_Tc2/1(q22)
  [q2] -> Bc2_Rot_B12/1(q2)
  [q21] -> Bc2_Rot_B32/1(q21)
  Bus Selector/2 -> [q21]  "<q21>"
  Bus Selector/1 -> [q22]  "<q22>"
  Bus Selector/3 -> [q2]  "<q2>"
  [geomPropRS2] -> Bus Selector/1  "geomPropRS2"
  [WRotXS1] -> Bus Selector1/1  "WRotXRS1"
  WRotXRS1/1 -> [WRotXS1]  "WRotXRS1"
  geomPropRS2/1 -> [geomPropRS2]  "geomPropRS2"
  [WRotXS2] -> WRotXRS2/1  "WRotXRS2"
  [rotMatsRS2] -> rotMatsRS2/1  "rotMatsRS2"
  Bus Creator1/1 -> [WRotXS2]  "WRotXRS2"
  [WRotB12] -> Bus Creator1/1  "W_Rot_B12"
  [WRotTc2] -> Bus Creator1/2  "W_Rot_Tc2"
  [WRotP22] -> Bus Creator1/3  "W_Rot_P22"
  [WRotB42] -> Bus Creator1/5  "W_Rot_B42"
  [WRotB32] -> Bus Creator1/4  "W_Rot_B32"
  [WRotB32] -> Product4/1  "W_Rot_B32"
  [B32RotB42] -> Product4/2  "B32_Rot_B42"
  Product4/1 -> [WRotB42]  "W_Rot_B42"
  Product3/1 -> [WRotB32]  "W_Rot_B32"
  [Bc2RotB32] -> Product3/2  "Bc2_Rot_B32"
  [WRotBc2] -> Product3/1  "W_Rot_Bc2"
  [WRotBc2] -> Product/1  "W_Rot_Bc2"
  Bus Selector1/1 -> [WRotBc2]  "<W_Rot_Bc2>"
  [WRotTc2] -> Product2/1  "W_Rot_Tc2"
  Product2/1 -> [WRotP22]  "W_Rot_P22"
  [Tc2RotP22] -> Product2/2  "Tc2_Rot_P22"
  [B12RotTc2] -> Product1/2  "B12_Rot_Tc2"
  Product1/1 -> [WRotTc2]  "W_Rot_Tc2"
  [WRotB12] -> Product1/1  "W_Rot_B12"
  Product/1 -> [WRotB12]  "W_Rot_B12"
  [Bc2RotB12] -> Product/2  "Bc2_Rot_B12"
  [Bc2RotB12] -> Bus Creator/6  "Bc2_Rot_B12"
  [B12RotTc2] -> Bus Creator/5  "B12_Rot_Tc2"
  [Bc2RotB32] -> Bus Creator/4  "Bc2_Rot_B32"
  [B32RotB42] -> Bus Creator/3  "B32_Rot_B42"
  [B42RotTc2] -> Bus Creator/2  "B42_Rot_Tc2"
  [Tc2RotP22] -> Bus Creator/1  "Tc2_Rot_P22"
  B42_Rot_Tc2/1(B42_Rot_Tc2) -> [B42RotTc2]  "B42_Rot_Tc2"
  B32_Rot_B42/1 -> [B32RotB42]  "B32_Rot_B42"
  Bc2_Rot_B32/1(Bc2_Rot_B32) -> [Bc2RotB32]  "Bc2_Rot_B32"
  B12_Rot_Tc2/1 -> [B12RotTc2]  "B12_Rot_Tc2"
  Bc2_Rot_B12/1(Bc2_Rot_B12) -> [Bc2RotB12]  "Bc2_Rot_B12"
  Tc2_Rot_P22/1 -> [Tc2RotP22]  "Tc2_Rot_P22"
  Bus Creator/1 -> [rotMatsRS2]  "rotMatsRS2"

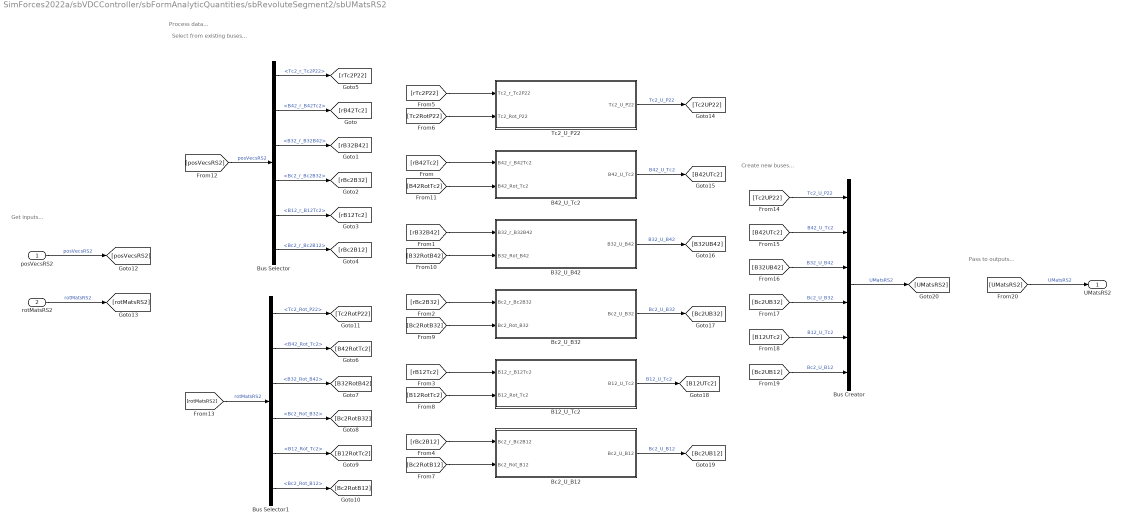
== system SimForces2022a/sbVDCController/sbFormAnalyticQuantities/sbRevoluteSegment2/sbUMatsRS2 ==
  note: Select from existing buses...
  note: Get inputs...
  note: Create new buses...
  note: Process data...
  note: Pass to outputs...
  posVecsRS2 : Inport
  rotMatsRS2 : Inport  Port=2
  B12_U_Tc2 : MATLAB Function  TreatAsAtomicUnit=on
  B32_U_B42 : MATLAB Function  TreatAsAtomicUnit=on
  B42_U_Tc2 : MATLAB Function  TreatAsAtomicUnit=on
  Bc2_U_B12 : MATLAB Function  TreatAsAtomicUnit=on
  Bc2_U_B32 : MATLAB Function  TreatAsAtomicUnit=on
  Bus Creator : BusCreator  Inputs=Tc2_U_P22,B42_U_Tc2,B32_U_B42,Bc2_U_B32,B12_U_Tc2,Bc2_U_B12
  Bus Selector : BusSelector  OutputSignals=Tc2_r_Tc2P22,B42_r_B42Tc2,B32_r_B32B42,Bc2_r_Bc2B32,B12_r_B12Tc2,Bc2_r_Bc2B12
  Bus Selector1 : BusSelector  OutputSignals=Tc2_Rot_P22,B42_Rot_Tc2,B32_Rot_B42,Bc2_Rot_B32,B12_Rot_Tc2,Bc2_Rot_B12
  Tc2_U_P22 : MATLAB Function  TreatAsAtomicUnit=on
  UMatsRS2 : Outport
  wires:
  [UMatsRS2] -> UMatsRS2/1  "UMatsRS2"
  Bus Creator/1 -> [UMatsRS2]  "UMatsRS2"
  [Bc2UB12] -> Bus Creator/6  "Bc2_U_B12"
  [B12UTc2] -> Bus Creator/5  "B12_U_Tc2"
  [Bc2UB32] -> Bus Creator/4  "Bc2_U_B32"
  [B32UB42] -> Bus Creator/3  "B32_U_B42"
  [B42UTc2] -> Bus Creator/2  "B42_U_Tc2"
  Bc2_U_B12/1(Bc2_U_B12) -> [Bc2UB12]  "Bc2_U_B12"
  B42_U_Tc2/1(B42_U_Tc2) -> [B42UTc2]  "B42_U_Tc2"
  B32_U_B42/1(B32_U_B42) -> [B32UB42]  "B32_U_B42"
  Bc2_U_B32/1(Bc2_U_B32) -> [Bc2UB32]  "Bc2_U_B32"
  B12_U_Tc2/1(B12_U_Tc2) -> [B12UTc2]  "B12_U_Tc2"
  [Tc2UP22] -> Bus Creator/1  "Tc2_U_P22"
  Tc2_U_P22/1(Tc2_U_P22) -> [Tc2UP22]  "Tc2_U_P22"
  [rotMatsRS2] -> Bus Selector1/1  "rotMatsRS2"
  [posVecsRS2] -> Bus Selector/1  "posVecsRS2"
  rotMatsRS2/1 -> [rotMatsRS2]  "rotMatsRS2"
  posVecsRS2/1 -> [posVecsRS2]  "posVecsRS2"
  [Tc2RotP22] -> Tc2_U_P22/2(Tc2_Rot_P22)
  [rTc2P22] -> Tc2_U_P22/1(Tc2_r_Tc2P22)
  Bus Selector1/1 -> [Tc2RotP22]  "<Tc2_Rot_P22>"
  Bus Selector/1 -> [rTc2P22]  "<Tc2_r_Tc2P22>"
  Bus Selector/2 -> [rB42Tc2]  "<B42_r_B42Tc2>"
  [rB42Tc2] -> B42_U_Tc2/1(B42_r_B42Tc2)
  Bus Selector/3 -> [rB32B42]  "<B32_r_B32B42>"
  Bus Selector/5 -> [rB12Tc2]  "<B12_r_B12Tc2>"
  Bus Selector/4 -> [rBc2B32]  "<Bc2_r_Bc2B32>"
  Bus Selector/6 -> [rBc2B12]  "<Bc2_r_Bc2B12>"
  [rBc2B12] -> Bc2_U_B12/1(Bc2_r_Bc2B12)
  [rB12Tc2] -> B12_U_Tc2/1(B12_r_B12Tc2)
  [rBc2B32] -> Bc2_U_B32/1(Bc2_r_Bc2B32)
  [rB32B42] -> B32_U_B42/1(B32_r_B32B42)
  Bus Selector1/2 -> [B42RotTc2]  "<B42_Rot_Tc2>"
  Bus Selector1/3 -> [B32RotB42]  "<B32_Rot_B42>"
  Bus Selector1/4 -> [Bc2RotB32]  "<Bc2_Rot_B32>"
  Bus Selector1/5 -> [B12RotTc2]  "<B12_Rot_Tc2>"
  Bus Selector1/6 -> [Bc2RotB12]  "<Bc2_Rot_B12>"
  [Bc2RotB12] -> Bc2_U_B12/2(Bc2_Rot_B12)
  [B12RotTc2] -> B12_U_Tc2/2(B12_Rot_Tc2)
  [Bc2RotB32] -> Bc2_U_B32/2(Bc2_Rot_B32)
  [B32RotB42] -> B32_U_B42/2(B32_Rot_B42)
  [B42RotTc2] -> B42_U_Tc2/2(B42_Rot_Tc2)

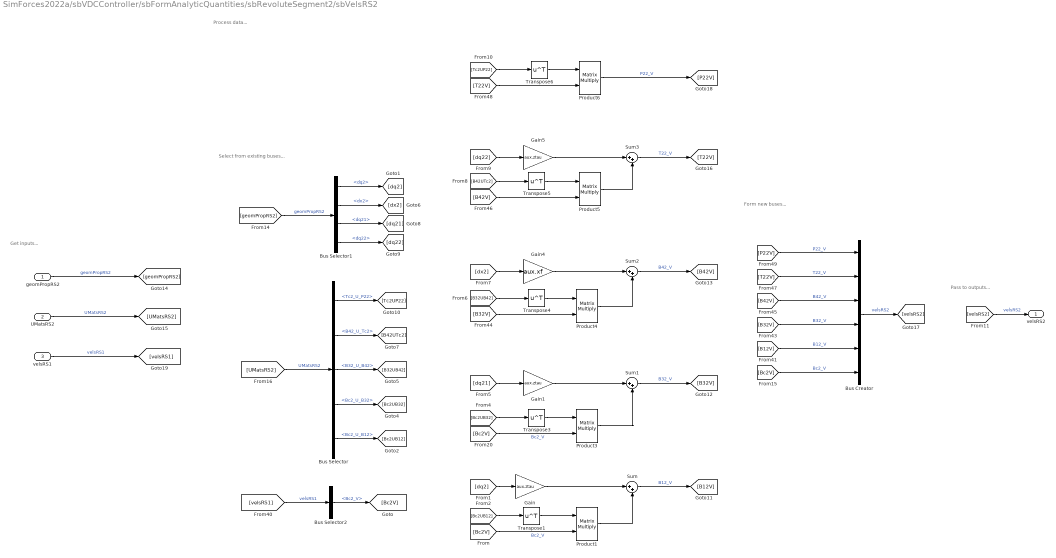
== system SimForces2022a/sbVDCController/sbFormAnalyticQuantities/sbRevoluteSegment2/sbVelsRS2 ==
  note: Get inputs...
  note: Select from existing buses...
  note: Form new buses...
  note: Process data...
  note: Pass to outputs...
  geomPropRS2 : Inport
  UMatsRS2 : Inport  Port=2
  velsRS1 : Inport  Port=3
  Bus Creator : BusCreator  Inputs=P22_V,T22_V,B42_V,B32_V,B12_V,Bc2_V
  Bus Selector : BusSelector  OutputSignals=Tc2_U_P22,B42_U_Tc2,B32_U_B42,Bc2_U_B32,Bc2_U_B12
  Bus Selector1 : BusSelector  OutputSignals=dq2,dx2,dq21,dq22
  Bus Selector2 : BusSelector  OutputSignals=Bc2_V
  Gain : Gain  Gain=aux.ztau
  Gain1 : Gain  Gain=aux.ztau
  Gain4 : Gain  Gain=aux.xf
  Gain5 : Gain  Gain=aux.ztau
  Product{1,3..6} (5 alike) : Product  Multiplication=Matrix(*)
  Sum{,1..3} (4 alike) : Sum  Inputs=|++
  Transpose{1,3..6} (5 alike) : Math  Operator=transpose
  velsRS2 : Outport
  wires:
  Product6/1 -> [P22V]  "P22_V"
  [velsRS2] -> velsRS2/1  "velsRS2"
  Bus Creator/1 -> [velsRS2]  "velsRS2"
  [P22V] -> Bus Creator/1  "P22_V"
  [T22V] -> Product6/2
  [T22V] -> Bus Creator/2  "T22_V"
  Sum3/1 -> [T22V]  "T22_V"
  [B42V] -> Bus Creator/3  "B42_V"
  [B42V] -> Product5/2
  Sum2/1 -> [B42V]  "B42_V"
  [B32V] -> Product4/2
  [B32V] -> Bus Creator/4  "B32_V"
  [B12V] -> Bus Creator/5  "B12_V"
  [Bc2V] -> Product3/2  "Bc2_V"
  [Bc2V] -> Product1/2  "Bc2_V"
  [Bc2V] -> Bus Creator/6  "Bc2_V"
  [geomPropRS2] -> Bus Selector1/1  "geomPropRS2"
  [UMatsRS2] -> Bus Selector/1  "UMatsRS2"
  [velsRS1] -> Bus Selector2/1  "velsRS1"
  velsRS1/1 -> [velsRS1]  "velsRS1"
  UMatsRS2/1 -> [UMatsRS2]  "UMatsRS2"
  geomPropRS2/1 -> [geomPropRS2]  "geomPropRS2"
  [Tc2UP22] -> Transpose6/1
  Transpose6/1 -> Product6/1
  Bus Selector/1 -> [Tc2UP22]  "<Tc2_U_P22>"
  Bus Selector2/1 -> [Bc2V]  "<Bc2_V>"
  Product1/1 -> Sum/2
  Sum/1 -> [B12V]  "B12_V"
  Gain1/1 -> Sum1/1
  Gain5/1 -> Sum3/1
  Gain/1 -> Sum/1
  Product4/1 -> Sum2/2
  Gain4/1 -> Sum2/1
  Product5/1 -> Sum3/2
  Transpose1/1 -> Product1/1
  Bus Selector1/1 -> [dq2]  "<dq2>"
  [dq2] -> Gain/1
  Bus Selector/5 -> [Bc2UB12]  "<Bc2_U_B12>"
  [Bc2UB12] -> Transpose1/1
  Bus Selector/4 -> [Bc2UB32]  "<Bc2_U_B32>"
  Transpose3/1 -> Product3/1
  [Bc2UB32] -> Transpose3/1
  Product3/1 -> Sum1/2
  [dq21] -> Gain1/1
  Bus Selector/3 -> [B32UB42]  "<B32_U_B42>"
  Transpose4/1 -> Product4/1
  [B32UB42] -> Transpose4/1
  Sum1/1 -> [B32V]  "B32_V"
  Bus Selector1/2 -> [dx2]  "<dx2>"
  [dx2] -> Gain4/1
  Bus Selector/2 -> [B42UTc2]  "<B42_U_Tc2>"
  [B42UTc2] -> Transpose5/1
  Transpose5/1 -> Product5/1
  Bus Selector1/4 -> [dq22]  "<dq22>"
  Bus Selector1/3 -> [dq21]  "<dq21>"
  [dq22] -> Gain5/1

== system SimForces2022a/sbVDCController/sbFormTotalRequiredForces/sbTotalRequiredForcesPS2/sbFilteredVelocityDerivativeB52 ==
  u : Inport
  Demux : Demux  Outputs=6
  Mux : Mux  Inputs=6
  sbDiscreteDerivative1 : Subsystem
  sbDiscreteDerivative2 : Subsystem
  sbDiscreteDerivative3 : Subsystem
  sbDiscreteDerivative4 : Subsystem
  sbDiscreteDerivative5 : Subsystem
  sbDiscreteDerivative6 : Subsystem
  sbLowPassFilter1 : Subsystem
  sbLowPassFilter2 : Subsystem
  sbLowPassFilter3 : Subsystem
  sbLowPassFilter4 : Subsystem
  sbLowPassFilter5 : Subsystem
  sbLowPassFilter6 : Subsystem
  du : Outport
  wires:
  Demux/3 -> sbDiscreteDerivative3/1(u)
  sbDiscreteDerivative5/1(du/dt) -> sbLowPassFilter5/1(dV)
  Mux/1 -> du/1
  Demux/4 -> sbDiscreteDerivative4/1(u)
  Demux/1 -> sbDiscreteDerivative1/1(u)
  sbLowPassFilter2/1(dVFilt) -> Mux/2
  Demux/6 -> sbDiscreteDerivative6/1(u)
  sbDiscreteDerivative1/1(du/dt) -> sbLowPassFilter1/1(dV)
  Demux/5 -> sbDiscreteDerivative5/1(u)
  Demux/2 -> sbDiscreteDerivative2/1(u)
  u/1 -> Demux/1
  sbLowPassFilter1/1(dVFilt) -> Mux/1
  sbDiscreteDerivative6/1(du/dt) -> sbLowPassFilter6/1(dV)
  sbLowPassFilter6/1(dVFilt) -> Mux/6
  sbDiscreteDerivative2/1(du/dt) -> sbLowPassFilter2/1(dV)
  sbDiscreteDerivative3/1(du/dt) -> sbLowPassFilter3/1(dV)
  sbLowPassFilter3/1(dVFilt) -> Mux/3
  sbLowPassFilter4/1(dVFilt) -> Mux/4
  sbDiscreteDerivative4/1(du/dt) -> sbLowPassFilter4/1(dV)
  sbLowPassFilter5/1(dVFilt) -> Mux/5

== system SimForces2022a/sbVDCController/sbFormTotalRequiredForces/sbTotalRequiredForcesPS2/sbFilteredVelocityDerivativeP22 ==
  u : Inport
  Demux : Demux  Outputs=6
  Mux : Mux  Inputs=6
  sbDiscreteDerivative1 : Subsystem
  sbDiscreteDerivative2 : Subsystem
  sbDiscreteDerivative3 : Subsystem
  sbDiscreteDerivative4 : Subsystem
  sbDiscreteDerivative5 : Subsystem
  sbDiscreteDerivative6 : Subsystem
  sbLowPassFilter1 : Subsystem
  sbLowPassFilter2 : Subsystem
  sbLowPassFilter3 : Subsystem
  sbLowPassFilter4 : Subsystem
  sbLowPassFilter5 : Subsystem
  sbLowPassFilter6 : Subsystem
  du : Outport
  wires:
  Demux/3 -> sbDiscreteDerivative3/1(u)
  sbDiscreteDerivative5/1(du/dt) -> sbLowPassFilter5/1(dV)
  Mux/1 -> du/1
  Demux/4 -> sbDiscreteDerivative4/1(u)
  Demux/1 -> sbDiscreteDerivative1/1(u)
  sbLowPassFilter2/1(dVFilt) -> Mux/2
  Demux/6 -> sbDiscreteDerivative6/1(u)
  sbDiscreteDerivative1/1(du/dt) -> sbLowPassFilter1/1(dV)
  Demux/5 -> sbDiscreteDerivative5/1(u)
  Demux/2 -> sbDiscreteDerivative2/1(u)
  u/1 -> Demux/1
  sbLowPassFilter1/1(dVFilt) -> Mux/1
  sbDiscreteDerivative6/1(du/dt) -> sbLowPassFilter6/1(dV)
  sbLowPassFilter6/1(dVFilt) -> Mux/6
  sbDiscreteDerivative2/1(du/dt) -> sbLowPassFilter2/1(dV)
  sbDiscreteDerivative3/1(du/dt) -> sbLowPassFilter3/1(dV)
  sbLowPassFilter3/1(dVFilt) -> Mux/3
  sbLowPassFilter4/1(dVFilt) -> Mux/4
  sbDiscreteDerivative4/1(du/dt) -> sbLowPassFilter4/1(dV)
  sbLowPassFilter5/1(dVFilt) -> Mux/5

== system SimForces2022a/sbVDCController/sbFormTotalRequiredForces/sbTotalRequiredForcesPS2/sbFilteredVelocityDerivativeP32 ==
  u : Inport
  Demux : Demux  Outputs=6
  Mux : Mux  Inputs=6
  sbDiscreteDerivative1 : Subsystem
  sbDiscreteDerivative2 : Subsystem
  sbDiscreteDerivative3 : Subsystem
  sbDiscreteDerivative4 : Subsystem
  sbDiscreteDerivative5 : Subsystem
  sbDiscreteDerivative6 : Subsystem
  sbLowPassFilter1 : Subsystem
  sbLowPassFilter2 : Subsystem
  sbLowPassFilter3 : Subsystem
  sbLowPassFilter4 : Subsystem
  sbLowPassFilter5 : Subsystem
  sbLowPassFilter6 : Subsystem
  du : Outport
  wires:
  Demux/3 -> sbDiscreteDerivative3/1(u)
  sbDiscreteDerivative5/1(du/dt) -> sbLowPassFilter5/1(dV)
  Mux/1 -> du/1
  Demux/4 -> sbDiscreteDerivative4/1(u)
  Demux/1 -> sbDiscreteDerivative1/1(u)
  sbLowPassFilter2/1(dVFilt) -> Mux/2
  Demux/6 -> sbDiscreteDerivative6/1(u)
  sbDiscreteDerivative1/1(du/dt) -> sbLowPassFilter1/1(dV)
  Demux/5 -> sbDiscreteDerivative5/1(u)
  Demux/2 -> sbDiscreteDerivative2/1(u)
  u/1 -> Demux/1
  sbLowPassFilter1/1(dVFilt) -> Mux/1
  sbDiscreteDerivative6/1(du/dt) -> sbLowPassFilter6/1(dV)
  sbLowPassFilter6/1(dVFilt) -> Mux/6
  sbDiscreteDerivative2/1(du/dt) -> sbLowPassFilter2/1(dV)
  sbDiscreteDerivative3/1(du/dt) -> sbLowPassFilter3/1(dV)
  sbLowPassFilter3/1(dVFilt) -> Mux/3
  sbLowPassFilter4/1(dVFilt) -> Mux/4
  sbDiscreteDerivative4/1(du/dt) -> sbLowPassFilter4/1(dV)
  sbLowPassFilter5/1(dVFilt) -> Mux/5
